simulink model "HH"  (Simulink 7.5)
settings: Solver=ode45  StartTime=0.0  StopTime=20.0  FixedStep=0.001  RelTol=1e-3
values from neighbouring files (symbols this model uses):
  Cm = 1e-6/1e-4    (= 0.01)    [modeloHH.m]
  GKmax = 36e-3    (= 0.036)    [modeloHH.m]
  GL = 0.3e-3    (= 0.0003)    [modeloHH.m]
  GNAmax = 120e-3    (= 0.12)    [modeloHH.m]
  VK = Vr - 12    (= -77)    [modeloHH.m]
  VL = Vr + 10.613    (= -54.387)    [modeloHH.m]
  VNA = Vr + 115    (= 50)    [modeloHH.m]
  Vr = -65    [modeloHH.m]
settings Model: Creator=Mariano  LastModifiedBy=Mariano

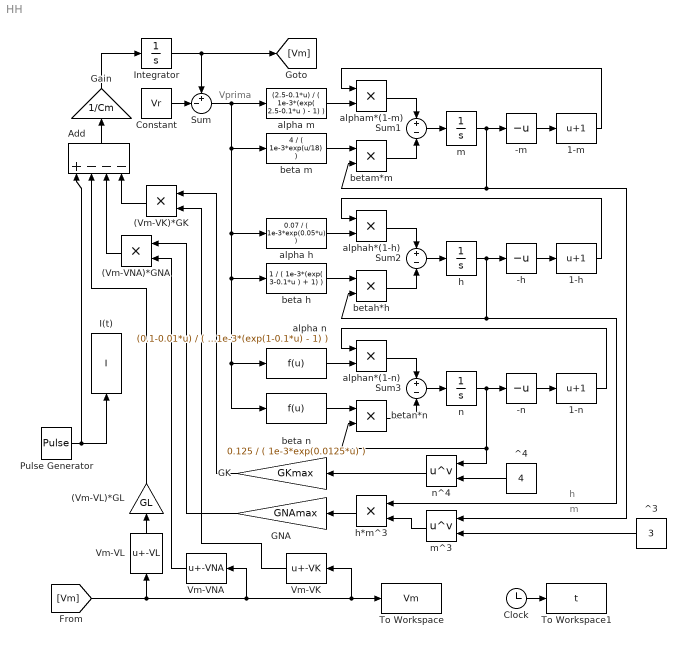
== system HH ==
  note: Vprima
  note: h
  note: m
  (Vm-VK)*GK : Product  OutDataType=fixdt(1, 16)  OutScaling=2^0  RndMeth=Zero
  (Vm-VL)*GL : Gain  Gain=GL  ParameterDataType=fixdt(1, 16)  ParameterScaling=2^0  OutDataType=fixdt(1, 16)  OutScaling=2^0
  (Vm-VNA)*GNA : Product  OutDataType=fixdt(1, 16)  OutScaling=2^0  RndMeth=Zero
  -h : UnaryMinus
  -m : UnaryMinus
  -n : UnaryMinus
  1-h : Bias  Bias=1
  1-m : Bias  Bias=1
  1-n : Bias  Bias=1
  Add : Sum  Inputs=+---  OutDataType=fixdt(1, 16)  OutScaling=2^-10
  Clock : Clock
      settings: Decimation=10
  Constant : Constant  Value=Vr  OutDataType=fixdt(1, 16)  OutScaling=2^0
  GK : Gain  Gain=GKmax  ParameterDataType=fixdt(1, 16)  ParameterScaling=2^0  OutDataType=fixdt(1, 16)  OutScaling=2^0
  GNA : Gain  Gain=GNAmax  ParameterDataType=fixdt(1, 16)  ParameterScaling=2^0  OutDataType=fixdt(1, 16)  OutScaling=2^0
  Gain : Gain  Gain=1/Cm  ParameterDataType=fixdt(1, 16)  ParameterScaling=2^0  OutDataType=fixdt(1, 16)  OutScaling=2^0
  I(t) : ToWorkspace  VariableName=I  SampleTime=-1  SaveFormat=Array
  Integrator : Integrator  InitialCondition=Vr
  Pulse Generator : DiscretePulseGenerator  PulseType=Time based  Amplitude=3  Period=2  PulseWidth=50  PhaseDelay=1  SampleTime=1
  Sum : Sum  Inputs=+-|  OutDataType=fixdt(1, 16)  OutScaling=2^0
  Sum1 : Sum  Inputs=+|-  OutDataType=fixdt(1, 16)  OutScaling=2^0
  Sum2 : Sum  Inputs=+|-  OutDataType=fixdt(1, 16)  OutScaling=2^0
  Sum3 : Sum  Inputs=+|-  OutDataType=fixdt(1, 16)  OutScaling=2^0
  To Workspace : ToWorkspace  VariableName=Vm  SampleTime=-1  SaveFormat=Array
  To Workspace1 : ToWorkspace  VariableName=t  SampleTime=-1  SaveFormat=Array
  Vm-VK : Bias  Bias=-VK
  Vm-VL : Bias  Bias=-VL
  Vm-VNA : Bias  Bias=-VNA
  ^3 : Constant  Value=3  OutDataType=fixdt(1, 16)  OutScaling=2^0
  ^4 : Constant  Value=4  OutDataType=fixdt(1, 16)  OutScaling=2^0
  alpha h : Fcn  Expr=0.07 / ( 1e-3*exp(0.05*u) )
  alpha m : Fcn  Expr=(2.5-0.1*u) / ( 1e-3*(exp( 2.5-0.1*u ) - 1) )
  alpha n : Fcn  Expr=(0.1-0.01*u) / ( 1e-3*(exp(1-0.1*u) - 1) )
  alphah*(1-h) : Product  OutDataType=fixdt(1, 16)  OutScaling=2^0  RndMeth=Zero
  alpham*(1-m) : Product  OutDataType=fixdt(1, 16)  OutScaling=2^0  RndMeth=Zero
  alphan*(1-n) : Product  OutDataType=fixdt(1, 16)  OutScaling=2^0  RndMeth=Zero
  beta h : Fcn  Expr=1 / ( 1e-3*(exp( 3-0.1*u ) + 1) )
  beta m : Fcn  Expr=4 / ( 1e-3*exp(u/18) )
  beta n : Fcn  Expr=0.125 / ( 1e-3*exp(0.0125*u) )
  betah*h : Product  OutDataType=fixdt(1, 16)  OutScaling=2^0  RndMeth=Zero
  betam*m : Product  OutDataType=fixdt(1, 16)  OutScaling=2^0  RndMeth=Zero
  betan*n : Product  OutDataType=fixdt(1, 16)  OutScaling=2^0  RndMeth=Zero
  h : Integrator  LimitOutput=on  UpperSaturationLimit=1  LowerSaturationLimit=0
  h*m^3 : Product  OutDataType=fixdt(1, 16)  OutScaling=2^0  RndMeth=Zero
  m : Integrator  LimitOutput=on  UpperSaturationLimit=1  LowerSaturationLimit=0
  m^3 : Math  Operator=pow  OutDataType=fixdt(1, 16)  OutScaling=2^0  SaturateOnIntegerOverflow=on
  n : Integrator  LimitOutput=on  UpperSaturationLimit=1  LowerSaturationLimit=0
  n^4 : Math  Operator=pow  OutDataType=fixdt(1, 16)  OutScaling=2^0  SaturateOnIntegerOverflow=on
  wires:
  Integrator/1 -> Sum/1, [Vm]
  Gain/1 -> Integrator/1
  Constant/1 -> Sum/2
  Sum/1 -> alpha m/1, beta m/1, alpha h/1, beta h/1, beta n/1, alpha n/1
  m/1 -> -m/1, betam*m/2, m^3/1
  -m/1 -> 1-m/1
  Sum1/1 -> m/1
  alpham*(1-m)/1 -> Sum1/1
  alpha m/1 -> alpham*(1-m)/2
  betam*m/1 -> Sum1/2
  beta m/1 -> betam*m/1
  1-m/1 -> alpham*(1-m)/1
  h/1 -> -h/1, betah*h/2, h*m^3/1
  -h/1 -> 1-h/1
  Sum2/1 -> h/1
  alphah*(1-h)/1 -> Sum2/1
  alpha h/1 -> alphah*(1-h)/2
  betah*h/1 -> Sum2/2
  beta h/1 -> betah*h/1
  1-h/1 -> alphah*(1-h)/1
  n/1 -> -n/1, betan*n/2, n^4/1
  -n/1 -> 1-n/1
  Sum3/1 -> n/1
  alphan*(1-n)/1 -> Sum3/1
  alpha n/1 -> alphan*(1-n)/2
  betan*n/1 -> Sum3/2
  beta n/1 -> betan*n/1
  1-n/1 -> alphan*(1-n)/1
  Add/1 -> Gain/1
  ^4/1 -> n^4/2
  ^3/1 -> m^3/2
  m^3/1 -> h*m^3/2
  (Vm-VK)*GK/1 -> Add/4
  (Vm-VNA)*GNA/1 -> Add/3
  (Vm-VL)*GL/1 -> Add/2
  n^4/1 -> GK/1
  [Vm] -> To Workspace/1, Vm-VK/1, Vm-VNA/1, Vm-VL/1
  h*m^3/1 -> GNA/1
  GK/1 -> (Vm-VK)*GK/1
  GNA/1 -> (Vm-VNA)*GNA/1
  Vm-VK/1 -> (Vm-VK)*GK/2
  Vm-VNA/1 -> (Vm-VNA)*GNA/2
  Vm-VL/1 -> (Vm-VL)*GL/1
  Pulse Generator/1 -> I(t)/1, Add/1
  Clock/1 -> To Workspace1/1
